simulink model "SlipControlV2_MTTE"  (R2015a)
settings: Solver=ode45  StartTime=0.0  StopTime=10.0  RelTol=1e-3
libraries: simulink x6
settings Model: Creator=Alexander  LastModifiedBy=Alexander

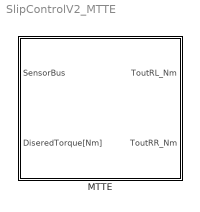
== system SlipControlV2_MTTE ==
  MTTE : Subsystem

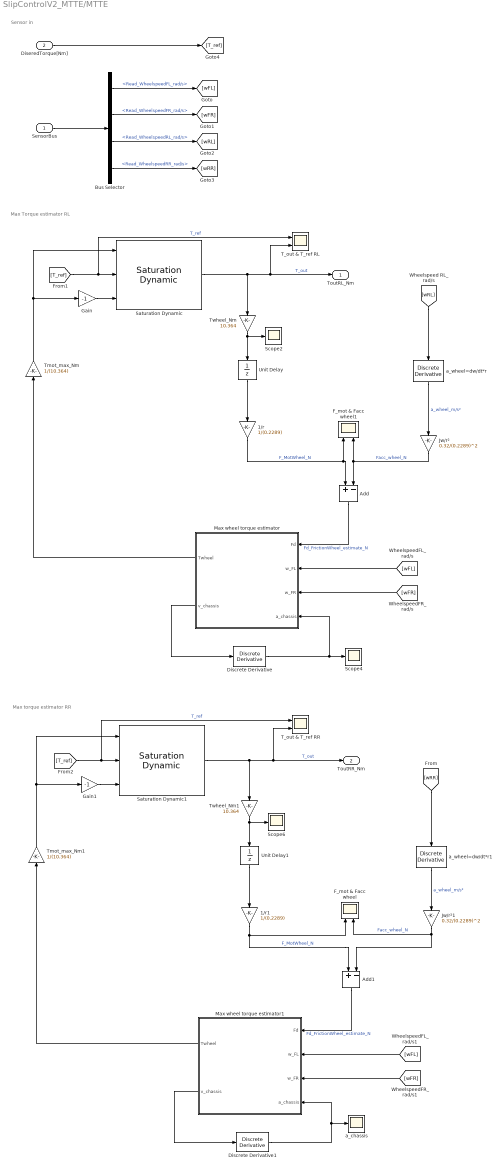
== system SlipControlV2_MTTE/MTTE ==
  note: Max torque estimator RR
  note: Max Torque estimator RL
  note: Sensor in
  SensorBus : Inport
  DiseredTorque[Nm] : Inport  Port=2
  1/r : Gain  Gain=1/(0.2289)
  1/r1 : Gain  Gain=1/(0.2289)
  Add : Sum  Inputs=+|-
  Add1 : Sum  Inputs=+|-
  Bus Selector : BusSelector  OutputSignals=Read_WheelspeedFL_rad/s,Read_WheelspeedFR_rad/s,Read_WheelspeedRL_rad/s,Read_WheelspeedRR_rad/s
  Discrete Derivative : simulink/Discrete/Discrete Derivative  gainval=1.0  ICPrevScaledInput=0.0  InputProcessing=Inherited  OutMin=[]  OutMax=[]  OutDataType=fixdt(1, 16)  OutScaling=2^-10  DoSatur=off
  Discrete Derivative1 : simulink/Discrete/Discrete Derivative  gainval=1.0  ICPrevScaledInput=0.0  InputProcessing=Inherited  OutMin=[]  OutMax=[]  OutDataType=fixdt(1, 16)  OutScaling=2^-10  DoSatur=off
  F_mot & Facc wheel : Scope  NumInputPorts=2
      settings: YMin=-300~-1755  YMax=600~1755  SaveName=ScopeData23
  F_mot & Facc wheel1 : Scope  NumInputPorts=2
      settings: YMin=-300~-1755  YMax=600~1755  SaveName=ScopeData18
  Gain : Gain  Gain=-1
  Gain1 : Gain  Gain=-1
  Jw/r² : Gain  Gain=0.32/(0.2289)^2
  Jw/r²1 : Gain  Gain=0.32/(0.2289)^2
  Max wheel torque estimator : MATLAB Function  TreatAsAtomicUnit=on
  Max wheel torque estimator1 : MATLAB Function  TreatAsAtomicUnit=on
  Saturation Dynamic : simulink/Discontinuities/Saturation Dynamic  OutMin=[]  OutMax=[]  OutDataTypeStr=Inherit: Same as second input  OutDataType=fixdt(1, 16)  OutScaling=2^-10  DoSatur=off
  Saturation Dynamic1 : simulink/Discontinuities/Saturation Dynamic  OutMin=[]  OutMax=[]  OutDataTypeStr=Inherit: Same as second input  OutDataType=fixdt(1, 16)  OutScaling=2^-10  DoSatur=off
  Scope2 : Scope
      settings: SaveName=ScopeData22
  Scope4 : Scope
      settings: YMin=-10  YMax=10  SaveName=ScopeData24
  Scope6 : Scope
      settings: SaveName=ScopeData26
  T_out & T_ref RL : Scope  NumInputPorts=2
      settings: YMin=-50~-50  YMax=50~50  SaveName=ScopeData17
  T_out & T_ref RR : Scope  NumInputPorts=2
      settings: YMin=-50~-50  YMax=50~50  SaveName=ScopeData28
  Tmot_max_Nm : Gain  Gain=1/(10.364)
  Tmot_max_Nm1 : Gain  Gain=1/(10.364)
  Twheel_Nm : Gain  Gain=10.364
  Twheel_Nm1 : Gain  Gain=10.364
  Unit Delay : UnitDelay  SampleTime=-1
  Unit Delay1 : UnitDelay  SampleTime=-1
  a_chassis : Scope
      settings: YMin=-10  YMax=10  SaveName=ScopeData27
  a_wheel=dw/dt*r : simulink/Discrete/Discrete Derivative  gainval=0.2289  ICPrevScaledInput=0.0  InputProcessing=Inherited  OutMin=[]  OutMax=[]  OutDataType=fixdt(1, 16)  OutScaling=2^-10  DoSatur=off
  a_wheel=dw/dt*r1 : simulink/Discrete/Discrete Derivative  gainval=0.2289  ICPrevScaledInput=0.0  InputProcessing=Inherited  OutMin=[]  OutMax=[]  OutDataType=fixdt(1, 16)  OutScaling=2^-10  DoSatur=off
  ToutRL_Nm : Outport
  ToutRR_Nm : Outport  Port=2
  wires:
  Unit Delay/1 -> 1/r/1
  a_wheel=dw/dt*r/1 -> Jw/r²/1  "a_wheel_m/s²"
  1/r/1 -> F_mot & Facc wheel1/1, Add/1  "F_MotWheel_N"
  Jw/r²/1 -> Add/2, F_mot & Facc wheel1/2  "Facc_wheel_N"
  Add/1 -> Max wheel torque estimator/1(Fd)  "Fd_FrictionWheel_estimate_N"
  Max wheel torque estimator/1(Twheel) -> Tmot_max_Nm/1
  [wFL] -> Max wheel torque estimator/2(w_FL)
  [wFR] -> Max wheel torque estimator/3(w_FR)
  Saturation Dynamic/1 -> ToutRL_Nm/1, T_out & T_ref RL/2, Twheel_Nm/1  "T_out"
  [T_ref] -> Saturation Dynamic/2, T_out & T_ref RL/1  "T_ref"
  Max wheel torque estimator/2(v_chassis) -> Discrete Derivative/1
  Discrete Derivative/1 -> Max wheel torque estimator/4(a_chassis), Scope4/1
  SensorBus/1 -> Bus Selector/1
  Bus Selector/1 -> [wFL]  "<Read_WheelspeedFL_rad/s>"
  Bus Selector/2 -> [wFR]  "<Read_WheelspeedFR_rad/s>"
  Bus Selector/3 -> [wRL]  "<Read_WheelspeedRL_rad/s>"
  [wRL] -> a_wheel=dw/dt*r/1
  Twheel_Nm/1 -> Scope2/1, Unit Delay/1
  Gain/1 -> Saturation Dynamic/3
  Tmot_max_Nm/1 -> Gain/1, Saturation Dynamic/1
  Unit Delay1/1 -> 1/r1/1
  a_wheel=dw/dt*r1/1 -> Jw/r²1/1  "a_wheel_m/s²"
  1/r1/1 -> F_mot & Facc wheel/1, Add1/1  "F_MotWheel_N"
  Jw/r²1/1 -> Add1/2, F_mot & Facc wheel/2  "Facc_wheel_N"
  Add1/1 -> Max wheel torque estimator1/1(Fd)  "Fd_FrictionWheel_estimate_N"
  Max wheel torque estimator1/1(Twheel) -> Tmot_max_Nm1/1
  [wFL] -> Max wheel torque estimator1/2(w_FL)
  [wFR] -> Max wheel torque estimator1/3(w_FR)
  Saturation Dynamic1/1 -> ToutRR_Nm/1, T_out & T_ref RR/2, Twheel_Nm1/1  "T_out"
  [T_ref] -> Saturation Dynamic1/2, T_out & T_ref RR/1  "T_ref"
  Max wheel torque estimator1/2(v_chassis) -> Discrete Derivative1/1
  Discrete Derivative1/1 -> Max wheel torque estimator1/4(a_chassis), a_chassis/1
  [wRR] -> a_wheel=dw/dt*r1/1
  Twheel_Nm1/1 -> Scope6/1, Unit Delay1/1
  Gain1/1 -> Saturation Dynamic1/3
  Tmot_max_Nm1/1 -> Gain1/1, Saturation Dynamic1/1
  Bus Selector/4 -> [wRR]  "<Read_WheelspeedRR_rad/s>"
  DiseredTorque[Nm]/1 -> [T_ref]

== matlab function SlipControlV2_MTTE/MTTE/Max wheel torque estimator1 ==
  data: Fd input; Twheel output; w_FL input; w_FR input; a_chassis input; v_chassis output
function [Twheel,v_chassis] = TorqueEstimation(Fd,w_FL,w_FR,a_chassis)
%% estimator wheel torque

Jw = 0.32; %[kgm²] Massatraagheid wiel (roterende componenten)
r=0.2286; %[m] straal wiel
a=0.9; %relacation factor a=Vchasis/Vwheel
M=302-70; %[kg] mass vehicle
m=70; %[kg] mass driver

w_chassis=(w_FL+w_FR)/2; % average speed
v_chassis=w_chassis*r; %[m/s] velocity of the chasis

Twheel = max(a_chassis*Jw/(a*r)+r*Fd,250);

== matlab function SlipControlV2_MTTE/MTTE/Max wheel torque estimator ==
  data: Fd input; Twheel output; w_FL input; w_FR input; a_chassis input; v_chassis output
function [Twheel,v_chassis] = TorqueEstimation(Fd,w_FL,w_FR,a_chassis)
%% estimator wheel torque

Jw = 0.32; %[kgm²] Massatraagheid wiel (roterende componenten)
r=0.2286; %[m] straal wiel
a=0.9; %relacation factor a=Vchasis/Vwheel
M=302-70; %[kg] mass vehicle
m=70; %[kg] mass driver

w_chassis=(w_FL+w_FR)/2; % average speed
v_chassis=w_chassis*r; %[m/s] velocity of the chasis

Twheel = max(a_chassis*Jw/(a*r)+r*Fd,250);
